simulink model "RTex"  (Simulink 6.6)
settings: Solver=ode3  StartTime=0.0  StopTime=inf  FixedStep=0.05  RelTol=1e-3
libraries: RT x1
settings Model: Creator=ugur  LastModifiedBy=ugur  SimulationMode=external  ExtModeTrigMode=oneshot  ExtModeArmWhenConnect=off
settings DataIOCC: LimitDataPoints=off
settings OptimizationCC: BlockReduction=off  BooleanDataType=off  LocalBlockOutputs=off
settings DebuggingCC: SignalResolutionControl=TryResolveAllWithWarning  SolverPrmCheckMsg=none  MultiTaskDSMMsg=warning  MultiTaskCondExecSysMsg=none  StrictBusMsg=None
settings HardwareCC: TargetEndianess=LittleEndian  TargetHWDeviceType=MATLAB Host  ProdEqTarget=off
settings RTWCC: MakeCommand="make_rtw S_FUNCTIONS_LIB=\"..\\winmm.lib ..\\rt.lib\""  RetainRTWFile=on  IncludeERTFirstTime=on
settings GRTTargetCC: ExtMode=on

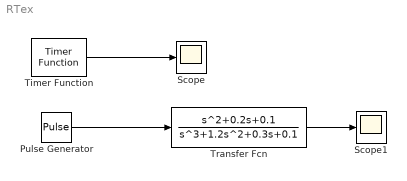
== system RTex ==
  Pulse Generator : DiscretePulseGenerator  PulseType=Time based  Period=1  PulseWidth=50
  Scope : Scope
      settings: YMin=0  YMax=50  SaveName=timing  DataFormat=Array
  Scope1 : Scope
      settings: YMin=0  YMax=0.65
  Timer Function : RT/Timer Function  step=50  tmrpriority=HIGH  ThPriority=TIME CRITICAL
  Transfer Fcn : TransferFcn  Numerator=[1 0.2 0.1]  Denominator=[1 1.2 0.3 0.1]
  wires:
  Timer Function/1 -> Scope/1
  Pulse Generator/1 -> Transfer Fcn/1
  Transfer Fcn/1 -> Scope1/1
